simulink model "MOSSE_HDL_final"  (Simulink 8.3)
settings: Solver=FixedStepDiscrete  SolverMode=SingleTasking  StartTime=0.0  StopTime=30*640*360  RelTol=1e-3
InitFcn:
  | %% DSPBuilder Start
  | alt_dspbuilder_update_model(bdroot)
  | %% DSPBuilder End
  | param
StopFcn:
  | % r = rcount.Data(:,:);
  | % w = wcount.Data(:,:);
  | % d = dout.Data(:,:);
  | % ir = read.Data(:,:);
  | % iw = write.Data(:,:);
  | % z = double([ir iw d r w]');
  | %logic_analyzer
values from neighbouring files (symbols this model uses):
  Gau = [4035 -3983 3832 -3589 3269 -2890 2472 -2039 1612 -1211 854 -553 ... (4096 elements, 1x4096)]    [Gauss_coeff.mat]    (also in param.m = reshape(conj(Gau'), 1, 4096))
undefined symbols (not defined in the file or in its folder): gray, psr, source_1, source_2, State_Machine, State_Transition_Table1, window_hann
libraries: allblocks_alteradspbuilder2 x166, hdlsllib x24, hdldemolib x3, simulink x2, dspsigattribs x2, dspmtrx3 x2, visionsinks x1, visiontextngfix x1, dspvision x1
(part 3 of 4)

== system MOSSE_HDL_final/DSP_Builder_Compute_PSR/Std1 ==
  finish_flag : Inport
  demul_sel : Inport  Port=2
  Input_data : Inport  Port=3
  mean_ena : Inport  Port=4
  mean : Inport  Port=5
  std_count_ena : Inport  Port=6
  std_reset : Inport  Port=7
  Barrel Shifter : allblocks_alteradspbuilder2/Barrel Shifter  BusType=Signed Integer  bwl=44  bwr=8  pipeline=off  infer_distance=off  distance_length=4  ShiftDirection=Shift right  use_ena=off  use_aclr=off  UseDedicatedCircuitry=off  pipeline_display=0  allowFloatingPointOverride=on  logOutputs=off  logFile=d:\Project\AutoTracking\model\MOSSE_work\MOSSE_model\MOSSE_Final_models\tb_MOSSE_HDL_final\MOSSE%5FHDL%5Ffinal_DSP%5FBuilder%5FCompute%5FPSR_Std1_Barrel+Shifter.fixedpointlog
  Bitwise Logical Bus Operator : allblocks_alteradspbuilder2/Bitwise Logical Bus Operator  BusType=Unsigned Integer  bwl=1  bwr=0  LogicalOperator=AND  pipeline_display=0
  Constant1 : allblocks_alteradspbuilder2/Constant  mask_cst=0  BusType=Signed Integer  bwl=32  bwr=0  roundMode=Truncate  satMode=Wrap  SpecifyClock=off  allowFloatingPointOverride=on  logOutputs=off  logFile=d:\Project\AutoTracking\model\MOSSE_work\MOSSE_model\MOSSE_Final_models\tb_MOSSE_HDL_final\MOSSE%5FHDL%5Ffinal_DSP%5FBuilder%5FCompute%5FPSR_Std1_Constant1.fixedpointlog
  Constant2 : allblocks_alteradspbuilder2/Constant  mask_cst=12  BusType=Unsigned Integer  bwl=4  bwr=0  roundMode=Truncate  satMode=Wrap  SpecifyClock=off  allowFloatingPointOverride=on  logOutputs=off  logFile=d:\Project\AutoTracking\model\MOSSE_work\MOSSE_model\MOSSE_Final_models\tb_MOSSE_HDL_final\MOSSE%5FHDL%5Ffinal_DSP%5FBuilder%5FCompute%5FPSR_Std1_Constant2.fixedpointlog
  Delay1 : allblocks_alteradspbuilder2/Delay  pipeline=1  pipeline_display=1  ClockPhase=1  use_ena=off  use_sclr=off  allowFloatingPointOverride=on  logOutputs=off  logFile=d:\Project\AutoTracking\model\MOSSE_work\MOSSE_model\MOSSE_Final_models\tb_MOSSE_HDL_final\MOSSE%5FHDL%5Ffinal_DSP%5FBuilder%5FCompute%5FPSR_Std1_Delay1.fixedpointlog  use_init=off  reset_value=1
  Delay2 : allblocks_alteradspbuilder2/Delay  pipeline=1  pipeline_display=1  ClockPhase=1  use_ena=off  use_sclr=off  allowFloatingPointOverride=on  logOutputs=off  logFile=d:\Project\AutoTracking\model\MOSSE_work\MOSSE_model\MOSSE_Final_models\tb_MOSSE_HDL_final\MOSSE%5FHDL%5Ffinal_DSP%5FBuilder%5FCompute%5FPSR_Std1_Delay2.fixedpointlog  use_init=off  reset_value=1
  Multiplexer : allblocks_alteradspbuilder2/Multiplexer  numInputs=2  pipeline=0  oneHot=off  pipeline_display=0  use_ena=off  use_aclr=off  allowFloatingPointOverride=on  logOutputs=off  logFile=d:\Project\AutoTracking\model\MOSSE_work\MOSSE_model\MOSSE_Final_models\tb_MOSSE_HDL_final\MOSSE%5FHDL%5Ffinal_DSP%5FBuilder%5FCompute%5FPSR_Std1_Multiplexer.fixedpointlog
  Multiplexer2 : allblocks_alteradspbuilder2/Multiplexer  numInputs=2  pipeline=0  oneHot=off  pipeline_display=0  use_ena=off  use_aclr=off  allowFloatingPointOverride=on  logOutputs=off  logFile=d:\Project\AutoTracking\model\MOSSE_work\MOSSE_model\MOSSE_Final_models\tb_MOSSE_HDL_final\MOSSE%5FHDL%5Ffinal_DSP%5FBuilder%5FCompute%5FPSR_Std1_Multiplexer2.fixedpointlog
  Pipelined Adder : allblocks_alteradspbuilder2/Pipelined Adder  BusType=Signed Integer  bwl=32  bwr=0  pipeline=0  pipeline_display=0  AddSubDirection=SUB  use_cin=off  use_ovl=off  use_addsub=off  use_ena=off  use_aclr=off  or_aclr_inputs=on
  Pipelined Adder2 : allblocks_alteradspbuilder2/Pipelined Adder  BusType=Signed Integer  bwl=44  bwr=0  pipeline=1  pipeline_display=1  AddSubDirection=ADD  use_cin=off  use_ovl=off  use_addsub=off  use_ena=off  use_aclr=on  or_aclr_inputs=off
  Product : allblocks_alteradspbuilder2/Product  BusType=Signed Integer  bwl=32  bwr=0  pipeline=0  pipeline_display=0  phase_selection=1  use_ena=off  use_aclr=off  UseLPM=off  UseDedicatedCircuitry=on  allowFloatingPointOverride=on  logOutputs=off  logFile=d:\Project\AutoTracking\model\MOSSE_work\MOSSE_model\MOSSE_Final_models\tb_MOSSE_HDL_final\MOSSE%5FHDL%5Ffinal_DSP%5FBuilder%5FCompute%5FPSR_Std1_Product.fixedpointlog
  Square Root : allblocks_alteradspbuilder2/Square Root  BusType=Unsigned Integer  bwl=44  bwr=0  pipeline=0  pipeline_display=0  use_remain=off  use_ena=off  use_aclr=off
  Std_finish : Outport
  Std_val : Outport  Port=2
  wires:
  Pipelined Adder/1 -> Product/2, Product/1
  Product/1 -> Pipelined Adder2/1
  Constant2/1 -> Barrel Shifter/2
  Pipelined Adder2/1 -> Pipelined Adder2/2, Barrel Shifter/1
  Barrel Shifter/1 -> Square Root/1
  Square Root/1 -> Multiplexer2/3
  Input_data/1 -> Pipelined Adder/1
  demul_sel/1 -> Bitwise Logical Bus Operator/2
  finish_flag/1 -> Bitwise Logical Bus Operator/1
  Delay1/1 -> Std_finish/1
  Constant1/1 -> Multiplexer/2
  mean_ena/1 -> Multiplexer/1
  mean/1 -> Multiplexer/3
  Multiplexer/1 -> Pipelined Adder/2
  std_count_ena/1 -> Multiplexer2/1
  Multiplexer2/1 -> Delay2/1
  Delay2/1 -> Std_val/1, Multiplexer2/2
  Bitwise Logical Bus Operator/1 -> Delay1/1
  std_reset/1 -> Pipelined Adder2/3

== system MOSSE_HDL_final/DSP_Builder_Compute_PSR/Vals_gen ==
  count_ena : Inport
  counter : Inport  Port=2
  demul_sel : Inport  Port=3
  Constant2 : allblocks_alteradspbuilder2/Constant  mask_cst=0  BusType=Single Bit  bwl=16  bwr=0  roundMode=Truncate  satMode=Wrap  SpecifyClock=off  allowFloatingPointOverride=on  logOutputs=off  logFile=d:\Project\AutoTracking\model\MOSSE_work\MOSSE_model\MOSSE_Final_models\tb_MOSSE_HDL_final\MOSSE%5FHDL%5Ffinal_DSP%5FBuilder%5FCompute%5FPSR_Vals%5Fgen_Constant2.fixedpointlog
  Demultiplexer : allblocks_alteradspbuilder2/Demultiplexer  numOutputs=2  pipeline_display=1  use_ena=off  use_sclr=off  allowFloatingPointOverride=on  logOutputs=off  logFile=d:\Project\AutoTracking\model\MOSSE_work\MOSSE_model\MOSSE_Final_models\tb_MOSSE_HDL_final\MOSSE%5FHDL%5Ffinal_DSP%5FBuilder%5FCompute%5FPSR_Vals%5Fgen_Demultiplexer%3A%3Aq.fixedpointlog,d:\Project\AutoTracking\model\MOSSE_work\MOSSE_model\MOSSE_Final_models\tb_MOSSE_HDL_final\MOSSE%5FHDL%5Ffinal_DSP%5FBuilder%5FCompute%5FPSR_Vals%5Fgen_Demultiplexer%3A%3Aq.fixedpointlog,
  Multiplexer : allblocks_alteradspbuilder2/Multiplexer  numInputs=2  pipeline=0  oneHot=off  pipeline_display=0  use_ena=off  use_aclr=off  allowFloatingPointOverride=on  logOutputs=off  logFile=d:\Project\AutoTracking\model\MOSSE_work\MOSSE_model\MOSSE_Final_models\tb_MOSSE_HDL_final\MOSSE%5FHDL%5Ffinal_DSP%5FBuilder%5FCompute%5FPSR_Vals%5Fgen_Multiplexer.fixedpointlog
  1_channel : Outport
  2_channel : Outport  Port=2
  wires:
  Multiplexer/1 -> Demultiplexer/1
  Demultiplexer/1 -> 1_channel/1
  Demultiplexer/2 -> 2_channel/1
  demul_sel/1 -> Demultiplexer/2
  Constant2/1 -> Multiplexer/2
  counter/1 -> Multiplexer/3
  count_ena/1 -> Multiplexer/1

== system MOSSE_HDL_final/DSP_Builder_Mult_complex/Gauss_table ==
  rst : Inport
  enb : Inport  Port=2
  Counter : allblocks_alteradspbuilder2/Counter  BusType=Unsigned Integer  bwl=12  bwr=0  use_modulo=off  modulo=255  SpecifyClock=off  direction=Increment  use_sload=off  use_sset=off  svalue=1  use_clk_ena=off  use_ena=on  use_sclr=on  pipeline_display=1
  ROM : allblocks_alteradspbuilder2/ROM  numwords=4096  BusType=Signed Integer  bwl=16  bwr=0  memory_type=AUTO  ram_type=ROM  initialization=From MATLAB array  init_file=input.hex  init_array=imag(Gau)  register_outputs=off  use_ena=off  ClockPhase=1  pipeline_display=1  allowFloatingPointOverride=on  logOutputs=off  logFile=E:\Work\ComputerVision\ObjectTrack\MOSSE\autotrackigproject\Model\MOSSE_algorithm\MOSSE_simulink\tb_MOSSE_HDL_final\MOSSE%5FHDL%5Ffinal_DSP%5FBuilder%5FMult%5Fcomplex_Gauss%5Ftable_ROM.fixedpointlog  enable_runtime_mod=off  instance_name=AAAA
  ROM1 : allblocks_alteradspbuilder2/ROM  numwords=4096  BusType=Signed Integer  bwl=16  bwr=0  memory_type=AUTO  ram_type=ROM  initialization=From MATLAB array  init_file=input.hex  init_array=real(Gau)  register_outputs=off  use_ena=off  ClockPhase=1  pipeline_display=1  allowFloatingPointOverride=on  logOutputs=off  logFile=E:\Work\ComputerVision\ObjectTrack\MOSSE\autotrackigproject\Model\MOSSE_algorithm\MOSSE_simulink\tb_MOSSE_HDL_final\MOSSE%5FHDL%5Ffinal_DSP%5FBuilder%5FMult%5Fcomplex_Gauss%5Ftable_ROM1.fixedpointlog  enable_runtime_mod=off  instance_name=AAAA
  Coeff_real : Outport
  Coeff_imag : Outport  Port=2
  wires:
  Counter/1 -> ROM/1, ROM1/1
  ROM1/1 -> Coeff_real/1
  ROM/1 -> Coeff_imag/1
  rst/1 -> Counter/2
  enb/1 -> Counter/1

== system MOSSE_HDL_final/HDL_CODER_Subsystem/Comp_Shift_code_Subsys ==
  Max_num : Inport
  iaclr : Inport  Port=2
  Comp_Shift_code : MATLAB Function
  dx : Outport
  dy : Outport  Port=2
  wires:
  Comp_Shift_code/2(dy) -> dy/1
  Comp_Shift_code/1(dx) -> dx/1
  Max_num/1 -> Comp_Shift_code/2(max_num)
  iaclr/1 -> Comp_Shift_code/1(iaclr)

== system MOSSE_HDL_final/HDL_CODER_Subsystem/Complex_2_real_imag ==
  H1 : Inport
  H2 : Inport  Port=2
  Complex to Real-Imag_H1 : ComplexToRealImag
  Complex to Real-Imag_H2 : ComplexToRealImag
  Terminator : Terminator
  Real_H1 : Outport
  Real_H2 : Outport  Port=2
  Imag_H1 : Outport  Port=3
  wires:
  Complex to Real-Imag_H2/2 -> Terminator/1
  Complex to Real-Imag_H1/1 -> Real_H1/1
  Complex to Real-Imag_H2/1 -> Real_H2/1
  Complex to Real-Imag_H1/2 -> Imag_H1/1
  H2/1 -> Complex to Real-Imag_H2/1
  H1/1 -> Complex to Real-Imag_H1/1

== system MOSSE_HDL_final/HDL_CODER_Subsystem/FFT2D_System ==
  en_R : Inport
  read_R : Inport  Port=2
  write_R : Inport  Port=3
  iData : Inport  Port=4
  iMux_mult : Inport  Port=5
  Corr_Data : Inport  Port=6
  Mux : Inport  Port=7
  image : Inport  Port=8
  Start : Inport  Port=9
  Enb : Inport  Port=10
  FFT2D_System : Subsystem
  Mux_Mult : Subsystem
  R_RAM : Subsystem
  F* : Outport
  F : Outport  Port=2
  IFFT_res : Outport  Port=3
  data_ready : Outport  Port=4
  end : Outport  Port=5
  wires:
  en_R/1 -> R_RAM/1(en_m)
  read_R/1 -> R_RAM/2(read_m)
  write_R/1 -> R_RAM/3(write_m)
  R_RAM/1(oData) -> FFT2D_System/1(Input1)
  image/1 -> FFT2D_System/3(Input2)
  Mux/1 -> FFT2D_System/2(Mux)
  Start/1 -> FFT2D_System/4(Start)
  Enb/1 -> FFT2D_System/5(Enb)
  FFT2D_System/2(data_ready) -> data_ready/1
  FFT2D_System/3(end) -> end/1
  iMux_mult/1 -> Mux_Mult/1(iMux_muLt)
  Corr_Data/1 -> Mux_Mult/2(Corr)
  FFT2D_System/1(oFFT2) -> Mux_Mult/3(iData)
  Mux_Mult/1(F*) -> F*/1
  Mux_Mult/2(F) -> F/1
  Mux_Mult/3(IFFT_res) -> IFFT_res/1
  iData/1 -> R_RAM/4(iData)

== system MOSSE_HDL_final/HDL_CODER_Subsystem/IFFT_MUX ==
  IFFT_res : Inport
  Mux : Inport  Port=2
  IFFT_res1 : Inport  Port=3
  Complex to Real-Imag2 : ComplexToRealImag  Output=Real  SampleTime=1
  Data Type Conversion2 : DataTypeConversion  OutDataTypeStr=int16
  IFFT_div : hdlsllib/HDL Operations/Bit Shift  mode=Shift Right Arithmetic  N=12
  IFFT_ress_mult : MultiPortSwitch  DataPortOrder=Zero-based contiguous  Inputs=2  zeroidx=on  SampleTime=1
  RAM_data : Outport
  oData : Outport  Port=2
  wires:
  Complex to Real-Imag2/1 -> IFFT_div/1
  IFFT_res1/1 -> IFFT_ress_mult/3
  Data Type Conversion2/1 -> RAM_data/1, IFFT_ress_mult/2
  IFFT_ress_mult/1 -> oData/1
  Mux/1 -> IFFT_ress_mult/1
  IFFT_div/1 -> Data Type Conversion2/1
  IFFT_res/1 -> Complex to Real-Imag2/1

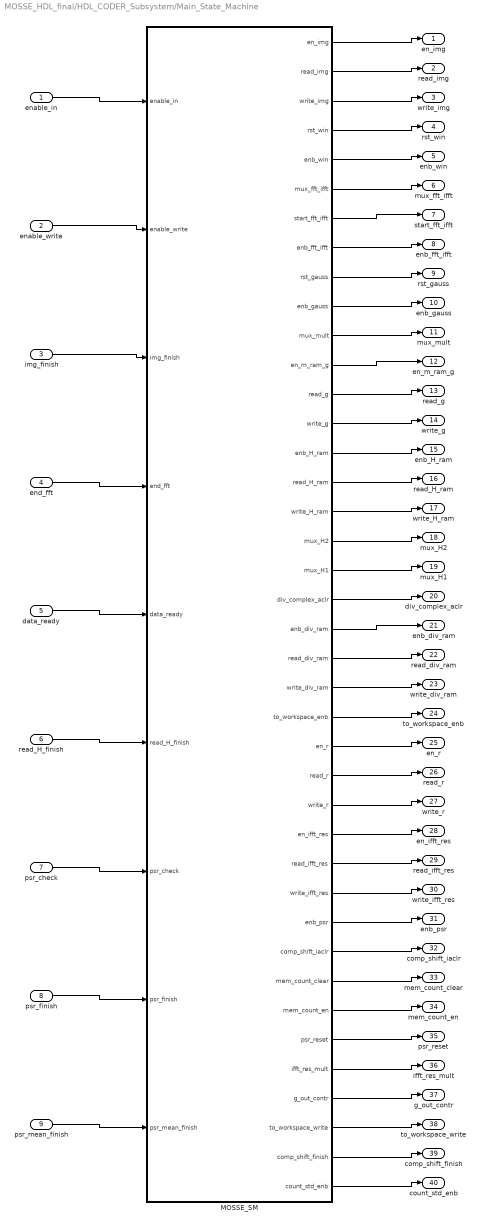
== system MOSSE_HDL_final/HDL_CODER_Subsystem/Main_State_Machine ==
  enable_in : Inport
  enable_write : Inport  Port=2
  img_finish : Inport  Port=3
  end_fft : Inport  Port=4
  data_ready : Inport  Port=5
  read_H_finish : Inport  Port=6
  psr_check : Inport  Port=7
  psr_finish : Inport  Port=8
  psr_mean_finish : Inport  Port=9
  MOSSE_SM : State Transition Table  TreatAsAtomicUnit=on
  en_img : Outport
  read_img : Outport  Port=2
  write_img : Outport  Port=3
  rst_win : Outport  Port=4
  enb_win : Outport  Port=5
  mux_fft_ifft : Outport  Port=6
  start_fft_ifft : Outport  Port=7
  enb_fft_ifft : Outport  Port=8
  rst_gauss : Outport  Port=9
  enb_gauss : Outport  Port=10
  mux_mult : Outport  Port=11
  en_m_ram_g : Outport  Port=12
  read_g : Outport  Port=13
  write_g : Outport  Port=14
  enb_H_ram : Outport  Port=15
  read_H_ram : Outport  Port=16
  write_H_ram : Outport  Port=17
  mux_H2 : Outport  Port=18
  mux_H1 : Outport  Port=19
  div_complex_aclr : Outport  Port=20
  enb_div_ram : Outport  Port=21
  read_div_ram : Outport  Port=22
  write_div_ram : Outport  Port=23
  to_workspace_enb : Outport  Port=24
  en_r : Outport  Port=25
  read_r : Outport  Port=26
  write_r : Outport  Port=27
  en_ifft_res : Outport  Port=28
  read_ifft_res : Outport  Port=29
  write_ifft_res : Outport  Port=30
  enb_psr : Outport  Port=31
  comp_shift_iaclr : Outport  Port=32
  mem_count_clear : Outport  Port=33
  mem_count_en : Outport  Port=34
  psr_reset : Outport  Port=35
  ifft_res_mult : Outport  Port=36
  g_out_contr : Outport  Port=37
  to_workspace_write : Outport  Port=38
  comp_shift_finish : Outport  Port=39
  count_std_enb : Outport  Port=40
  wires:
  MOSSE_SM/24(to_workspace_enb) -> to_workspace_enb/1
  MOSSE_SM/10(enb_gauss) -> enb_gauss/1
  MOSSE_SM/7(start_fft_ifft) -> start_fft_ifft/1
  MOSSE_SM/2(read_img) -> read_img/1
  MOSSE_SM/11(mux_mult) -> mux_mult/1
  MOSSE_SM/15(enb_H_ram) -> enb_H_ram/1
  img_finish/1 -> MOSSE_SM/3(img_finish)
  MOSSE_SM/6(mux_fft_ifft) -> mux_fft_ifft/1
  data_ready/1 -> MOSSE_SM/5(data_ready)
  MOSSE_SM/8(enb_fft_ifft) -> enb_fft_ifft/1
  MOSSE_SM/12(en_m_ram_g) -> en_m_ram_g/1
  MOSSE_SM/17(write_H_ram) -> write_H_ram/1
  MOSSE_SM/18(mux_H2) -> mux_H2/1
  MOSSE_SM/14(write_g) -> write_g/1
  MOSSE_SM/16(read_H_ram) -> read_H_ram/1
  enable_in/1 -> MOSSE_SM/1(enable_in)
  MOSSE_SM/13(read_g) -> read_g/1
  MOSSE_SM/4(rst_win) -> rst_win/1
  MOSSE_SM/5(enb_win) -> enb_win/1
  end_fft/1 -> MOSSE_SM/4(end_fft)
  MOSSE_SM/3(write_img) -> write_img/1
  MOSSE_SM/9(rst_gauss) -> rst_gauss/1
  MOSSE_SM/22(read_div_ram) -> read_div_ram/1
  MOSSE_SM/19(mux_H1) -> mux_H1/1
  MOSSE_SM/23(write_div_ram) -> write_div_ram/1
  MOSSE_SM/21(enb_div_ram) -> enb_div_ram/1
  MOSSE_SM/20(div_complex_aclr) -> div_complex_aclr/1
  read_H_finish/1 -> MOSSE_SM/6(read_H_finish)
  MOSSE_SM/25(en_r) -> en_r/1
  MOSSE_SM/1(en_img) -> en_img/1
  MOSSE_SM/26(read_r) -> read_r/1
  MOSSE_SM/27(write_r) -> write_r/1
  MOSSE_SM/28(en_ifft_res) -> en_ifft_res/1
  MOSSE_SM/29(read_ifft_res) -> read_ifft_res/1
  MOSSE_SM/34(mem_count_en) -> mem_count_en/1
  MOSSE_SM/31(enb_psr) -> enb_psr/1
  MOSSE_SM/30(write_ifft_res) -> write_ifft_res/1
  MOSSE_SM/32(comp_shift_iaclr) -> comp_shift_iaclr/1
  MOSSE_SM/33(mem_count_clear) -> mem_count_clear/1
  MOSSE_SM/36(ifft_res_mult) -> ifft_res_mult/1
  psr_check/1 -> MOSSE_SM/7(psr_check)
  psr_finish/1 -> MOSSE_SM/8(psr_finish)
  psr_mean_finish/1 -> MOSSE_SM/9(psr_mean_finish)
  MOSSE_SM/35(psr_reset) -> psr_reset/1
  MOSSE_SM/37(g_out_contr) -> g_out_contr/1
  enable_write/1 -> MOSSE_SM/2(enable_write)
  MOSSE_SM/38(to_workspace_write) -> to_workspace_write/1
  MOSSE_SM/39(comp_shift_finish) -> comp_shift_finish/1
  MOSSE_SM/40(count_std_enb) -> count_std_enb/1

== system MOSSE_HDL_final/HDL_CODER_Subsystem/Memory_Counter_Subsys ==
  dx : Inport
  dy : Inport  Port=2
  clear : Inport  Port=3
  en : Inport  Port=4
  Memory Counter : MATLAB Function
  addr : Outport
  wires:
  dy/1 -> Memory Counter/4(dy)
  en/1 -> Memory Counter/2(en)
  dx/1 -> Memory Counter/3(dx)
  clear/1 -> Memory Counter/1(clear)
  Memory Counter/1(count) -> addr/1

== system MOSSE_HDL_final/HDL_CODER_Subsystem/Mux_system ==
  iMux_Mult : Inport
  iData1 : Inport  Port=2
  iData2 : Inport  Port=3
  iH1_1 : Inport  Port=4
  iMux_H1 : Inport  Port=5
  iH1_2 : Inport  Port=6
  iMux_H2 : Inport  Port=7
  iH2_2 : Inport  Port=8
  iH2_1 : Inport  Port=9
  Delay2 : Delay  DelayLength=1  InitialCondition=0
  Delay3 : Delay  DelayLength=1  InitialCondition=0
  Mux_H1 : MultiPortSwitch  DataPortOrder=Zero-based contiguous  Inputs=2  zeroidx=on  SampleTime=1
  Mux_H2 : MultiPortSwitch  DataPortOrder=Zero-based contiguous  Inputs=2  zeroidx=on  SampleTime=1
  Mux_Mult1 : MultiPortSwitch  DataPortOrder=Zero-based contiguous  Inputs=2  zeroidx=on  SampleTime=1
  Mux_Mult2 : MultiPortSwitch  DataPortOrder=Zero-based contiguous  Inputs=2  zeroidx=on  SampleTime=1
  H2 : Outport
  H1 : Outport  Port=2
  oData1 : Outport  Port=3
  oData2 : Outport  Port=4
  wires:
  iH2_2/1 -> Mux_H2/3
  iH1_2/1 -> Mux_H1/3
  iMux_H2/1 -> Mux_H2/1
  iMux_H1/1 -> Mux_H1/1
  Mux_Mult1/1 -> oData1/1
  Mux_Mult2/1 -> oData2/1
  iData1/1 -> Delay3/1, Mux_Mult1/2
  Delay3/1 -> Mux_Mult1/3
  iData2/1 -> Mux_Mult2/2, Delay2/1
  Delay2/1 -> Mux_Mult2/3
  iMux_Mult/1 -> Mux_Mult1/1, Mux_Mult2/1
  Mux_H1/1 -> H1/1
  Mux_H2/1 -> H2/1
  iH1_1/1 -> Mux_H1/2
  iH2_1/1 -> Mux_H2/2

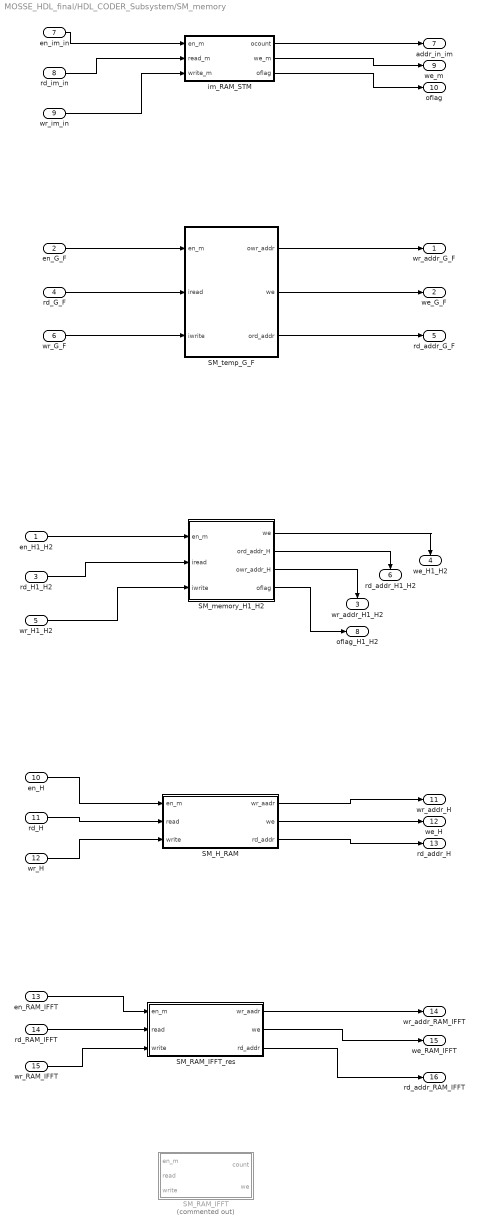
== system MOSSE_HDL_final/HDL_CODER_Subsystem/SM_memory ==
  en_H1_H2 : Inport
  en_G_F : Inport  Port=2
  rd_H1_H2 : Inport  Port=3
  rd_G_F : Inport  Port=4
  wr_H1_H2 : Inport  Port=5
  wr_G_F : Inport  Port=6
  en_im_in : Inport  Port=7
  rd_im_in : Inport  Port=8
  wr_im_in : Inport  Port=9
  en_H : Inport  Port=10
  rd_H : Inport  Port=11
  wr_H : Inport  Port=12
  en_RAM_IFFT : Inport  Port=13
  rd_RAM_IFFT : Inport  Port=14
  wr_RAM_IFFT : Inport  Port=15
  SM_H_RAM : Subsystem
  SM_RAM_IFFT : Subsystem  Commented=on
  SM_RAM_IFFT_res : Subsystem
  SM_memory_H1_H2 : Subsystem
  SM_temp_G_F : Subsystem
  im_RAM_STM : Subsystem
  wr_addr_G_F : Outport
  we_G_F : Outport  Port=2
  wr_addr_H1_H2 : Outport  Port=3
  we_H1_H2 : Outport  Port=4
  rd_addr_G_F : Outport  Port=5
  rd_addr_H1_H2 : Outport  Port=6
  addr_in_im : Outport  Port=7
  oflag_H1_H2 : Outport  Port=8
  we_m : Outport  Port=9
  oflag : Outport  Port=10
  wr_addr_H : Outport  Port=11
  we_H : Outport  Port=12
  rd_addr_H : Outport  Port=13
  wr_addr_RAM_IFFT : Outport  Port=14
  we_RAM_IFFT : Outport  Port=15
  rd_addr_RAM_IFFT : Outport  Port=16
  wires:
  en_im_in/1 -> im_RAM_STM/1(en_m)
  rd_im_in/1 -> im_RAM_STM/2(read_m)
  wr_im_in/1 -> im_RAM_STM/3(write_m)
  im_RAM_STM/1(ocount) -> addr_in_im/1
  im_RAM_STM/2(we_m) -> we_m/1
  im_RAM_STM/3(oflag) -> oflag/1
  en_RAM_IFFT/1 -> SM_RAM_IFFT_res/1(en_m)
  rd_RAM_IFFT/1 -> SM_RAM_IFFT_res/2(read)
  wr_RAM_IFFT/1 -> SM_RAM_IFFT_res/3(write)
  SM_RAM_IFFT_res/1(wr_aadr) -> wr_addr_RAM_IFFT/1
  SM_RAM_IFFT_res/2(we) -> we_RAM_IFFT/1
  en_H/1 -> SM_H_RAM/1(en_m)
  rd_H/1 -> SM_H_RAM/2(read)
  wr_H/1 -> SM_H_RAM/3(write)
  SM_H_RAM/1(wr_aadr) -> wr_addr_H/1
  SM_H_RAM/2(we) -> we_H/1
  SM_H_RAM/3(rd_addr) -> rd_addr_H/1
  SM_memory_H1_H2/1(we) -> we_H1_H2/1
  SM_memory_H1_H2/3(owr_addr_H) -> wr_addr_H1_H2/1
  SM_memory_H1_H2/2(ord_addr_H) -> rd_addr_H1_H2/1
  en_H1_H2/1 -> SM_memory_H1_H2/1(en_m)
  rd_H1_H2/1 -> SM_memory_H1_H2/2(iread)
  wr_H1_H2/1 -> SM_memory_H1_H2/3(iwrite)
  SM_memory_H1_H2/4(oflag) -> oflag_H1_H2/1
  SM_temp_G_F/3(ord_addr) -> rd_addr_G_F/1
  SM_temp_G_F/2(we) -> we_G_F/1
  SM_temp_G_F/1(owr_addr) -> wr_addr_G_F/1
  en_G_F/1 -> SM_temp_G_F/1(en_m)
  rd_G_F/1 -> SM_temp_G_F/2(iread)
  wr_G_F/1 -> SM_temp_G_F/3(iwrite)
  SM_RAM_IFFT_res/3(rd_addr) -> rd_addr_RAM_IFFT/1

== system MOSSE_HDL_final/HDL_CODER_Subsystem/psr_code_subsys ==
  enb : Inport
  rst : Inport  Port=2
  idata : Inport  Port=3
  count_std_enb : Inport  Port=4
  Compute_PSR_code : MATLAB Function
  counter : Outport
  max_index : Outport  Port=2
  max_value : Outport  Port=3
  mean_value : Outport  Port=4
  mean_finish : Outport  Port=5
  psr_finish : Outport  Port=6
  std_value : Outport  Port=7
  wires:
  Compute_PSR_code/6(mean_finish) -> mean_finish/1
  Compute_PSR_code/1(counter) -> counter/1
  Compute_PSR_code/4(mean_value) -> mean_value/1
  Compute_PSR_code/5(std_value) -> std_value/1
  Compute_PSR_code/2(max_index) -> max_index/1
  Compute_PSR_code/3(max_value) -> max_value/1
  Compute_PSR_code/7(psr_finish) -> psr_finish/1
  enb/1 -> Compute_PSR_code/1(enb)
  rst/1 -> Compute_PSR_code/2(rst)
  idata/1 -> Compute_PSR_code/3(idata)
  count_std_enb/1 -> Compute_PSR_code/4(count_std_enb)

== system MOSSE_HDL_final/Source/source_1 ==
  In1 : Inport
  Enable : EnablePort
  source_1 : LookupNDDirect  NumberOfTableDimensions=1  Table=source_1  TableDataTypeStr=int16
  Out1 : Outport
  wires:
  source_1/1 -> Out1/1
  In1/1 -> source_1/1

== system MOSSE_HDL_final/Source/source_2 ==
  In1 : Inport
  Enable : EnablePort
  source_2 : LookupNDDirect  NumberOfTableDimensions=1  Table=source_2  TableDataTypeStr=int16
  Out1 : Outport
  wires:
  source_2/1 -> Out1/1
  In1/1 -> source_2/1

== system MOSSE_HDL_final/Video_TestBench/Write_control_subsys ==
  addr_x : Inport
  addr_y : Inport  Port=2
  dx : Inport  Port=3
  dy : Inport  Port=4
  x_init : Inport  Port=5
  y_init : Inport  Port=6
  comp_shift_finish : Inport  Port=7
  Write_control_STM : State Transition Table  TreatAsAtomicUnit=on
  x_coord : Outport
  y_coord : Outport  Port=2
  enable_write : Outport  Port=3
  to_workspace_enb : Outport  Port=4
  frame_num : Outport  Port=5
  wires:
  x_init/1 -> Write_control_STM/6(x_init)
  y_init/1 -> Write_control_STM/7(y_init)
  dx/1 -> Write_control_STM/3(dx)
  dy/1 -> Write_control_STM/4(dy)
  Write_control_STM/1(x_coord) -> x_coord/1
  Write_control_STM/3(enable_write) -> enable_write/1
  Write_control_STM/2(y_coord) -> y_coord/1
  comp_shift_finish/1 -> Write_control_STM/5(comp_shift_finish)
  Write_control_STM/4(to_workspace_enable) -> to_workspace_enb/1
  addr_x/1 -> Write_control_STM/1(addr_x)
  addr_y/1 -> Write_control_STM/2(addr_y)
  Write_control_STM/5(frame_num) -> frame_num/1

== system MOSSE_HDL_final/Video_TestBench/deserialize1 ==
  serialin : Inport
  Buffer : Buffer  N=640*360  TreatMby1Signals=One channel
  Convert 1-D to 2-D : dspsigattribs/Convert 1-D to 2-D  M=640  N=360  frameBasedOut=off
  Frame Conversion : FrameConversion  OutFrame=Sample-based
  Transpose : dspmtrx3/Transpose  Hermitian=off  overflowFlag=on
  imgout : Outport
  wires:
  Buffer/1 -> Frame Conversion/1
  serialin/1 -> Buffer/1
  Convert 1-D to 2-D/1 -> Transpose/1
  Frame Conversion/1 -> Convert 1-D to 2-D/1
  Transpose/1 -> imgout/1

== system MOSSE_HDL_final/Video_TestBench/serialize ==
  img : Inport
  Convert 2-D to 1-D : dspsigattribs/Convert 2-D to 1-D
  Frame Conversion : FrameConversion
  Transpose : dspmtrx3/Transpose  Hermitian=off  overflowFlag=on
  Unbuffer : Unbuffer  SampleBasedProcessing=Same as frame based
  serial : Outport  SampleTime=1
  wires:
  Convert 2-D to 1-D/1 -> Frame Conversion/1
  img/1 -> Transpose/1
  Transpose/1 -> Convert 2-D to 1-D/1
  Frame Conversion/1 -> Unbuffer/1
  Unbuffer/1 -> serial/1

== system MOSSE_HDL_final/HDL_CODER_Subsystem/FFT2D_System/FFT2D_System ==
  Input1 : Inport
  Mux : Inport  Port=2
  Input2 : Inport  Port=3
  Start : Inport  Port=4
  Enb : Inport  Port=5
  Data Type Conversion1 : DataTypeConversion  OutDataTypeStr=fixdt(1,24,0)
  FFT/IFTT Mux : MultiPortSwitch  DataPortOrder=Zero-based contiguous  Inputs=2  zeroidx=on  OutDataTypeStr=fixdt(1,24,0)  SampleTime=1
  FFT2D/IFFT2D : Subsystem
  Real-Imag to Complex1 : RealImagToComplex  Input=Real  SampleTime=1
  oFFT2 : Outport
  data_ready : Outport  Port=2
  end : Outport  Port=3
  wires:
  FFT/IFTT Mux/1 -> FFT2D/IFFT2D/1(input)
  FFT2D/IFFT2D/3(end) -> end/1
  FFT2D/IFFT2D/1(oFFT2) -> oFFT2/1
  Input2/1 -> Data Type Conversion1/1
  Mux/1 -> FFT/IFTT Mux/1
  Enb/1 -> FFT2D/IFFT2D/3(Enb)
  Input1/1 -> FFT/IFTT Mux/2
  Data Type Conversion1/1 -> Real-Imag to Complex1/1
  Start/1 -> FFT2D/IFFT2D/2(Start)
  FFT2D/IFFT2D/2(data_ready) -> data_ready/1
  Real-Imag to Complex1/1 -> FFT/IFTT Mux/3

== system MOSSE_HDL_final/HDL_CODER_Subsystem/FFT2D_System/Mux_Mult ==
  iMux_muLt : Inport
  Corr : Inport  Port=2
  iData : Inport  Port=3
  Complex to Real-Imag : ComplexToRealImag
  Data Type Conversion3 : DataTypeConversion  OutDataTypeStr=int32
  Math Function1 : Math  Operator=conj  SaturateOnIntegerOverflow=on
  Mux_Mult : MultiPortSwitch  DataPortOrder=Zero-based contiguous  Inputs=2  zeroidx=on  SampleTime=1
  Real-Imag to Complex : RealImagToComplex
  Window_div1 : hdlsllib/HDL Operations/Bit Shift  mode=Shift Right Arithmetic  N=3
  Window_div2 : hdlsllib/HDL Operations/Bit Shift  mode=Shift Right Arithmetic  N=3
  F* : Outport
  F : Outport  Port=2
  IFFT_res : Outport  Port=3
  wires:
  Corr/1 -> Mux_Mult/3
  Math Function1/1 -> Mux_Mult/2
  iMux_muLt/1 -> Mux_Mult/1
  Data Type Conversion3/1 -> Complex to Real-Imag/1, IFFT_res/1
  Mux_Mult/1 -> F*/1
  iData/1 -> Data Type Conversion3/1
  Complex to Real-Imag/2 -> Window_div2/1
  Complex to Real-Imag/1 -> Window_div1/1
  Real-Imag to Complex/1 -> F/1, Math Function1/1
  Window_div1/1 -> Real-Imag to Complex/1
  Window_div2/1 -> Real-Imag to Complex/2

== system MOSSE_HDL_final/HDL_CODER_Subsystem/FFT2D_System/R_RAM ==
  en_m : Inport
  read_m : Inport  Port=2
  write_m : Inport  Port=3
  iData : Inport  Port=4
  Data Type Conversion : DataTypeConversion  OutDataTypeStr=fixdt(1,24,0)
  Math Function : Math  Operator=conj  SaturateOnIntegerOverflow=on
  Read_Write_SM6 : State Transition Table  TreatAsAtomicUnit=on
  Simple Dual Port RAM : hdlsllib/HDL Operations/Simple Dual Port RAM  ram_size=12
  WRADDR_R : hdlsllib/HDL Operations/HDL Counter  CountType=Free running  CountInit=0  CountStep=1  CountMax=100  CountFromType=Initial value  CountFrom=0  CountResetPort=on  CountLoadPort=off  CountEnbPort=on  CountDirPort=off  CountDataType=Unsigned  CountWordLen=12  CountFracLen=0  CountSampTime=1
  oData : Outport
  wires:
  Read_Write_SM6/3(enb_img) -> WRADDR_R/2
  write_m/1 -> Read_Write_SM6/3(write)
  en_m/1 -> Read_Write_SM6/1(en_m)
  read_m/1 -> Read_Write_SM6/2(read)
  Simple Dual Port RAM/1 -> oData/1
  Read_Write_SM6/2(rst_img) -> WRADDR_R/1
  Math Function/1 -> Data Type Conversion/1
  iData/1 -> Math Function/1
  Data Type Conversion/1 -> Simple Dual Port RAM/1
  WRADDR_R/1 -> Simple Dual Port RAM/4, Simple Dual Port RAM/2
  Read_Write_SM6/1(we) -> Simple Dual Port RAM/3

== system MOSSE_HDL_final/HDL_CODER_Subsystem/SM_memory/SM_H_RAM ==
  en_m : Inport
  read : Inport  Port=2
  write : Inport  Port=3
  RADDR_H2 : hdlsllib/HDL Operations/HDL Counter  CountType=Free running  CountInit=0  CountStep=1  CountMax=100  CountFromType=Initial value  CountFrom=0  CountResetPort=on  CountLoadPort=off  CountEnbPort=on  CountDirPort=off  CountDataType=Unsigned  CountWordLen=12  CountFracLen=0  CountSampTime=1
  Read_Write_SM1_patched_2 : State Transition Table  TreatAsAtomicUnit=on
  WADDR_H2 : hdlsllib/HDL Operations/HDL Counter  CountType=Free running  CountInit=0  CountStep=1  CountMax=100  CountFromType=Initial value  CountFrom=0  CountResetPort=on  CountLoadPort=off  CountEnbPort=on  CountDirPort=off  CountDataType=Unsigned  CountWordLen=12  CountFracLen=0  CountSampTime=1
  wr_aadr : Outport
  we : Outport  Port=2
  rd_addr : Outport  Port=3
  wires:
  RADDR_H2/1 -> rd_addr/1
  Read_Write_SM1_patched_2/2(rst_r) -> RADDR_H2/1
  Read_Write_SM1_patched_2/3(enb_r) -> RADDR_H2/2
  Read_Write_SM1_patched_2/5(enb_w) -> WADDR_H2/2
  Read_Write_SM1_patched_2/4(rst_w) -> WADDR_H2/1
  read/1 -> Read_Write_SM1_patched_2/2(read)
  Read_Write_SM1_patched_2/1(we) -> we/1
  en_m/1 -> Read_Write_SM1_patched_2/1(en_m)
  write/1 -> Read_Write_SM1_patched_2/3(write)
  WADDR_H2/1 -> wr_aadr/1

== system MOSSE_HDL_final/HDL_CODER_Subsystem/SM_memory/SM_RAM_IFFT ==
  en_m : Inport
  read : Inport  Port=2
  write : Inport  Port=3
  IFFT_counter : hdldemolib/HDL Counter  CountType=Free running  CountInit=0  CountStep=1  CountMax=100  CountFromType=Initial value  CountFrom=0  CountResetPort=on  CountLoadPort=off  CountEnbPort=on  CountDirPort=off  CountDataType=Unsigned  CountWordLen=12  CountFracLen=0  CountSampTime=1
  Read_Write_SM7 : State Transition Table  TreatAsAtomicUnit=on
  count : Outport
  we : Outport  Port=2
  wires:
  IFFT_counter/1 -> count/1
  Read_Write_SM7/2(rst_img) -> IFFT_counter/1
  Read_Write_SM7/3(enb_img) -> IFFT_counter/2
  Read_Write_SM7/1(we) -> we/1
  read/1 -> Read_Write_SM7/2(read)
  write/1 -> Read_Write_SM7/3(write)
  en_m/1 -> Read_Write_SM7/1(en_m)

== system MOSSE_HDL_final/HDL_CODER_Subsystem/SM_memory/SM_RAM_IFFT_res ==
  en_m : Inport
  read : Inport  Port=2
  write : Inport  Port=3
  RADDR_H2 : hdlsllib/HDL Operations/HDL Counter  CountType=Free running  CountInit=0  CountStep=1  CountMax=100  CountFromType=Initial value  CountFrom=0  CountResetPort=on  CountLoadPort=off  CountEnbPort=on  CountDirPort=off  CountDataType=Unsigned  CountWordLen=12  CountFracLen=0  CountSampTime=1
  Read_Write_SM1_patched_2 : State Transition Table  TreatAsAtomicUnit=on
  WADDR_H2 : hdlsllib/HDL Operations/HDL Counter  CountType=Free running  CountInit=0  CountStep=1  CountMax=100  CountFromType=Initial value  CountFrom=0  CountResetPort=on  CountLoadPort=off  CountEnbPort=on  CountDirPort=off  CountDataType=Unsigned  CountWordLen=12  CountFracLen=0  CountSampTime=1
  wr_aadr : Outport
  we : Outport  Port=2
  rd_addr : Outport  Port=3
  wires:
  RADDR_H2/1 -> rd_addr/1
  Read_Write_SM1_patched_2/2(rst_r) -> RADDR_H2/1
  Read_Write_SM1_patched_2/3(enb_r) -> RADDR_H2/2
  Read_Write_SM1_patched_2/5(enb_w) -> WADDR_H2/2
  Read_Write_SM1_patched_2/4(rst_w) -> WADDR_H2/1
  read/1 -> Read_Write_SM1_patched_2/2(read)
  Read_Write_SM1_patched_2/1(we) -> we/1
  en_m/1 -> Read_Write_SM1_patched_2/1(en_m)
  write/1 -> Read_Write_SM1_patched_2/3(write)
  WADDR_H2/1 -> wr_aadr/1

== system MOSSE_HDL_final/HDL_CODER_Subsystem/SM_memory/SM_memory_H1_H2 ==
  en_m : Inport
  iread : Inport  Port=2
  iwrite : Inport  Port=3
  Compare To Constant1 : simulink/Logic and Bit Operations/Compare To Constant  relop===  const=4095  OutDataTypeStr=boolean
  RADDR_H1 : hdlsllib/HDL Operations/HDL Counter  CountType=Free running  CountInit=0  CountStep=1  CountMax=100  CountFromType=Initial value  CountFrom=0  CountResetPort=on  CountLoadPort=off  CountEnbPort=on  CountDirPort=off  CountDataType=Unsigned  CountWordLen=12  CountFracLen=0  CountSampTime=1
  Read_Write_SM1_patched_1 : State Transition Table  TreatAsAtomicUnit=on
  WADDR_H1 : hdlsllib/HDL Operations/HDL Counter  CountType=Free running  CountInit=0  CountStep=1  CountMax=100  CountFromType=Initial value  CountFrom=0  CountResetPort=on  CountLoadPort=off  CountEnbPort=on  CountDirPort=off  CountDataType=Unsigned  CountWordLen=12  CountFracLen=0  CountSampTime=1
  we : Outport
  ord_addr_H : Outport  Port=2
  owr_addr_H : Outport  Port=3
  oflag : Outport  Port=4
  wires:
  iwrite/1 -> Read_Write_SM1_patched_1/3(write)
  Read_Write_SM1_patched_1/3(enb_r) -> RADDR_H1/2
  iread/1 -> Read_Write_SM1_patched_1/2(read)
  Read_Write_SM1_patched_1/2(rst_r) -> RADDR_H1/1
  Read_Write_SM1_patched_1/5(enb_w) -> WADDR_H1/2
  en_m/1 -> Read_Write_SM1_patched_1/1(en_m)
  Read_Write_SM1_patched_1/4(rst_w) -> WADDR_H1/1
  Compare To Constant1/1 -> oflag/1
  WADDR_H1/1 -> owr_addr_H/1
  Read_Write_SM1_patched_1/1(we) -> we/1
  RADDR_H1/1 -> Compare To Constant1/1, ord_addr_H/1

== system MOSSE_HDL_final/HDL_CODER_Subsystem/SM_memory/SM_temp_G_F ==
  en_m : Inport
  iread : Inport  Port=2
  iwrite : Inport  Port=3
  RDADDR_H_n : hdlsllib/HDL Operations/HDL Counter  CountType=Free running  CountInit=0  CountStep=1  CountMax=100  CountFromType=Initial value  CountFrom=0  CountResetPort=on  CountLoadPort=off  CountEnbPort=on  CountDirPort=off  CountDataType=Unsigned  CountWordLen=12  CountFracLen=0  CountSampTime=1
  Read_Write_SM1_patched_2 : State Transition Table  TreatAsAtomicUnit=on
  WRADDR_H_n : hdlsllib/HDL Operations/HDL Counter  CountType=Free running  CountInit=0  CountStep=1  CountMax=100  CountFromType=Initial value  CountFrom=0  CountResetPort=on  CountLoadPort=off  CountEnbPort=on  CountDirPort=off  CountDataType=Unsigned  CountWordLen=12  CountFracLen=0  CountSampTime=1
  owr_addr : Outport
  we : Outport  Port=2
  ord_addr : Outport  Port=3
  wires:
  WRADDR_H_n/1 -> owr_addr/1
  iread/1 -> Read_Write_SM1_patched_2/2(read)
  Read_Write_SM1_patched_2/1(we) -> we/1
  iwrite/1 -> Read_Write_SM1_patched_2/3(write)
  en_m/1 -> Read_Write_SM1_patched_2/1(en_m)
  RDADDR_H_n/1 -> ord_addr/1
  Read_Write_SM1_patched_2/2(rst_r) -> RDADDR_H_n/1
  Read_Write_SM1_patched_2/3(enb_r) -> RDADDR_H_n/2
  Read_Write_SM1_patched_2/4(rst_w) -> WRADDR_H_n/1
  Read_Write_SM1_patched_2/5(enb_w) -> WRADDR_H_n/2

== system MOSSE_HDL_final/HDL_CODER_Subsystem/SM_memory/im_RAM_STM ==
  en_m : Inport
  read_m : Inport  Port=2
  write_m : Inport  Port=3
  ADDR_iPix1 : hdlsllib/HDL Operations/HDL Counter  CountType=Free running  CountInit=0  CountStep=1  CountMax=100  CountFromType=Initial value  CountFrom=0  CountResetPort=on  CountLoadPort=off  CountEnbPort=on  CountDirPort=off  CountDataType=Unsigned  CountWordLen=14  CountFracLen=0  CountSampTime=1
  Compare To Constant : simulink/Logic and Bit Operations/Compare To Constant  relop===  const=16383  OutDataTypeStr=boolean
  Delay2 : Delay  DelayLength=1  InitialCondition=0
  Read_Write_patched_2 : State Transition Table  TreatAsAtomicUnit=on
  Terminator1 : Terminator
  Terminator2 : Terminator
  ocount : Outport
  we_m : Outport  Port=2
  oflag : Outport  Port=3
  wires:
  Compare To Constant/1 -> Delay2/1
  write_m/1 -> Read_Write_patched_2/3(write)
  Read_Write_patched_2/1(we) -> we_m/1
  read_m/1 -> Read_Write_patched_2/2(read)
  en_m/1 -> Read_Write_patched_2/1(en_m)
  ADDR_iPix1/1 -> ocount/1, Compare To Constant/1
  Read_Write_patched_2/4(rst_w) -> ADDR_iPix1/1
  Read_Write_patched_2/5(enb_w) -> ADDR_iPix1/2
  Read_Write_patched_2/2(rst_r) -> Terminator1/1
  Read_Write_patched_2/3(enb_r) -> Terminator2/1
  Delay2/1 -> oflag/1

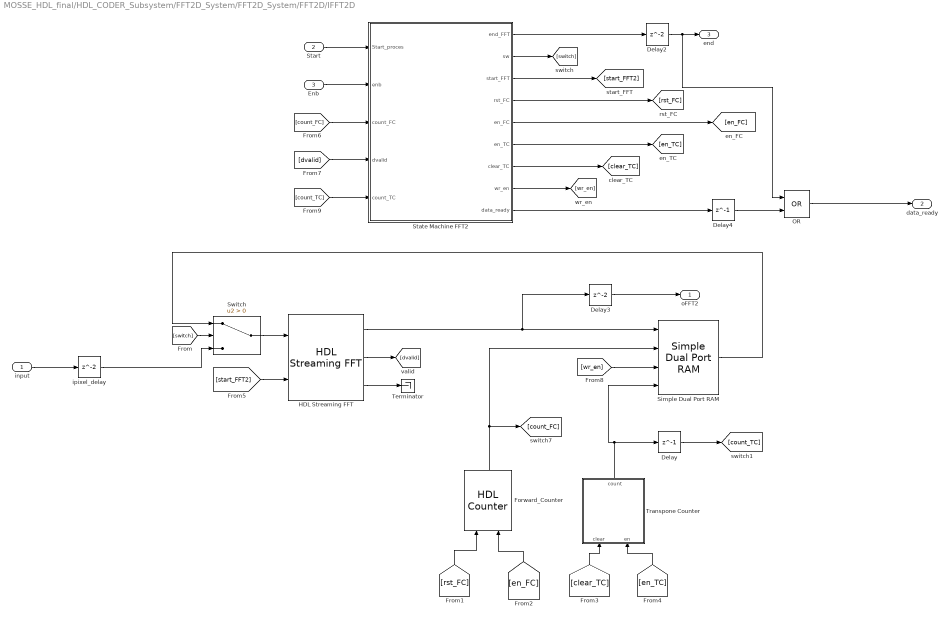
== system MOSSE_HDL_final/HDL_CODER_Subsystem/FFT2D_System/FFT2D_System/FFT2D/IFFT2D ==
  input : Inport
  Start : Inport  Port=2
  Enb : Inport  Port=3
  Delay : Delay  DelayLength=1  InitialCondition=0
  Delay2 : Delay  InitialCondition=0
  Delay3 : Delay  InitialCondition=0
  Delay4 : Delay  DelayLength=1  InitialCondition=0
  Forward_Counter : hdlsllib/HDL Operations/HDL Counter  CountType=Free running  CountInit=0  CountStep=1  CountMax=4095  CountFromType=Initial value  CountFrom=0  CountResetPort=on  CountLoadPort=off  CountEnbPort=on  CountDirPort=off  CountDataType=Unsigned  CountWordLen=12  CountFracLen=0  CountSampTime=1
  HDL Streaming FFT : hdldemolib/HDL Streaming FFT  N=64  rnd=Floor  sat=Wrap  sinemode=Same word length as input  sineWL=16  prodmode=Same as input  prodWL=32  prodFL=23  accumode=Same as input  accuWL=32  accuFL=0  outputmode=Same as input  outputWL=16  outputFL=8  isBitReversed=off  dispDelay=on
  OR : Logic  Operator=OR  IconShape=distinctive  AllPortsSameDT=off  OutDataTypeStr=boolean
  Simple Dual Port RAM : hdlsllib/HDL Operations/Simple Dual Port RAM  ram_size=12
  State Machine FFT2 : State Transition Table  TreatAsAtomicUnit=on
      settings: RTWSystemCode=Inline
  Switch : Switch  Criteria=u2 > Threshold  SampleTime=1
  Terminator : Terminator
  Transpone Counter : MATLAB Function
  ipixel_delay : Delay  InitialCondition=0  SampleTime=1
  oFFT2 : Outport
  data_ready : Outport  Port=2  OutDataTypeStr=boolean
  end : Outport  Port=3  OutDataTypeStr=boolean
  wires:
  HDL Streaming FFT/3 -> Terminator/1
  ipixel_delay/1 -> Switch/3
  HDL Streaming FFT/1 -> Delay3/1, Simple Dual Port RAM/1
  Switch/1 -> HDL Streaming FFT/1
  input/1 -> ipixel_delay/1
  State Machine FFT2/1(end_FFT) -> Delay2/1
  [switch] -> Switch/2
  State Machine FFT2/2(sw) -> [switch]
  State Machine FFT2/3(start_FFT) -> [start_FFT2]
  State Machine FFT2/4(rst_FC) -> [rst_FC]
  State Machine FFT2/5(en_FC) -> [en_FC]
  State Machine FFT2/6(en_TC) -> [en_TC]
  State Machine FFT2/7(clear_TC) -> [clear_TC]
  State Machine FFT2/8(wr_en) -> [wr_en]
  Start/1 -> State Machine FFT2/1(Start_proces)
  Enb/1 -> State Machine FFT2/2(enb)
  [clear_TC] -> Transpone Counter/1(clear)
  [en_TC] -> Transpone Counter/2(en)
  [start_FFT2] -> HDL Streaming FFT/2
  HDL Streaming FFT/2 -> [dvalid]
  [count_FC] -> State Machine FFT2/3(count_FC)
  [dvalid] -> State Machine FFT2/4(dvalid)
  [wr_en] -> Simple Dual Port RAM/3
  Forward_Counter/1 -> [count_FC], Simple Dual Port RAM/2
  [en_FC] -> Forward_Counter/2
  [rst_FC] -> Forward_Counter/1
  Simple Dual Port RAM/1 -> Switch/1
  [count_TC] -> State Machine FFT2/5(count_TC)
  Delay/1 -> [count_TC]
  Transpone Counter/1(count) -> Simple Dual Port RAM/4, Delay/1
  Delay2/1 -> OR/1, end/1
  Delay3/1 -> oFFT2/1
  Delay4/1 -> OR/2
  State Machine FFT2/9(data_ready) -> Delay4/1
  OR/1 -> data_ready/1

== matlab function HDL_CODER_Subsystem/psr_code_subsys/Compute_PSR_code ==
  data: counter output double; enb input double; rst input double; max_index output double; max_value output double; mean_value output double; std_value output double; mean_finish output double; psr_finish output double; idata input double; count_std_enb input double
function [counter, max_index, max_value, mean_value, std_value, mean_finish, psr_finish]  = psr(enb, rst, idata, count_std_enb)

numtype_idata = numerictype(1,16,0);
numtype_ind = numerictype(0,13,0);
numtype_temp = numerictype(1,44,0);
numtype_bool = numerictype(0,1,0);

numtype_fm = fimath('OverflowMode', 'saturate', 'RoundMode', 'zero');
persistent max_val max_ind temp mean_val std_val count max_mean_flag std_flag psr_flag mean_end psr_end

if isempty(max_val)
    max_val = fi(0, numtype_idata, numtype_fm);
end

if isempty(max_ind)
    max_ind = fi(0, numtype_ind, numtype_fm);
end

if isempty(count)
    count = fi(0, numtype_ind, numtype_fm);
end

if isempty(count_std_enb)
    count_std_enb = fi(0, numtype_bool, numtype_fm);
end

if isempty(temp)
    temp = fi(0, numtype_temp, numtype_fm);
end

if isempty(mean_val)
    mean_val = fi(0, numtype_idata, numtype_fm);
end

if isempty(std_val)
    std_val = fi(0, numtype_temp, numtype_fm);
end

if isempty(max_mean_flag)
    max_mean_flag = fi(0, numtype_bool, numtype_fm);
end

if isempty(std_flag)
    std_flag = fi(0, numtype_bool, numtype_fm);
end

if isempty(psr_flag)
    psr_flag = fi(0, numtype_bool, numtype_fm);
end

if isempty(mean_end)
    mean_end = fi(0, numtype_bool, numtype_fm);
end

if isempty(psr_end)
    psr_end = fi(0, numtype_bool, numtype_fm);
end

if rst
    max_val = fi(0, numtype_idata, numtype_fm);
    max_ind = fi(0, numtype_ind, numtype_fm);
    count = fi(0, numtype_ind, numtype_fm);
    temp = fi(0, numtype_temp, numtype_fm);
    mean_val = fi(0, numtype_idata, numtype_fm);
    std_val = fi(0, numtype_temp, numtype_fm);
    max_mean_flag = fi(1, numtype_bool, numtype_fm);
    std_flag = fi(0, numtype_bool, numtype_fm);
    psr_flag = fi(0, numtype_bool, numtype_fm);
    mean_end = fi(0, numtype_bool, numtype_fm);
    psr_end = fi(0, numtype_bool, numtype_fm);
    
elseif enb
    if max_mean_flag
        if idata > max_val
            max_val = fi(idata, numtype_idata, numtype_fm);
            max_ind = fi(count, numtype_ind, numtype_fm);
        end
        temp = fi(temp + idata, numtype_temp, numtype_fm);
        count = fi(count + 1, numtype_ind, numtype_fm);
        if count > 4096
            mean_val = fi(bitshift(temp, -12), numtype_idata, numtype_fm);
            temp = fi(0, numtype_temp, numtype_fm);
            count = fi(0, numtype_ind, numtype_fm);
            max_mean_flag = fi(0, numtype_bool, numtype_fm);
            std_flag = fi(1, numtype_bool, numtype_fm);
            mean_end = fi(1, numtype_bool, numtype_fm);
        end
    elseif count_std_enb
        if std_flag
            temp = fi((temp + (idata - mean_val)*(idata - mean_val)), numtype_temp, numtype_fm);
            count = fi(count + 1, numtype_ind, numtype_fm);
            if count > 4096        
                std_val = fi(bitshift(temp, -12), numtype_temp, numtype_fm);
                count = fi(0, numtype_ind, numtype_fm);
                std_flag = fi(0, numtype_bool, numtype_fm);
                psr_flag = fi(1, numtype_bool, numtype_fm);
            end
        elseif psr_flag
            count = fi(count + 1, numtype_ind, numtype_fm);
            if count > 6
                count = fi(0, numtype_ind, numtype_fm);
                psr_end = fi(1, numtype_bool, numtype_fm);
                psr_flag = fi(0, numtype_bool, numtype_fm);
            end
        end
    end       
end

counter = count;
max_index = max_ind;
max_value = max_val;
mean_value = mean_val;
std_value = std_val;
mean_finish = mean_end;
psr_finish = psr_end;

end

== matlab function HDL_CODER_Subsystem/FFT2D_System/FFT2D_System/FFT2D//IFFT2D/Transpone Counter ==
  data: count output fixdt(0,12,0); clear input double; en input double
function count  = count(clear, en)


result_nt = numerictype(0,12,0);
count_nt = numerictype(0,6,0);

result_fm = fimath('OverflowMode', 'saturate', 'RoundMode', 'floor');
n = fi(64, 0,7,0, result_fm);
persistent count_reg column row

if isempty(count_reg)
    count_reg = fi(0, result_nt, result_fm);
end

if isempty(column)
    column = fi(0, count_nt, result_fm);
end

if isempty(row)
    row = fi(0, count_nt, result_fm);
end


if clear
    row = fi(0, count_nt, result_fm);
    column = fi(0, count_nt, result_fm);
    count_reg = fi(0, result_nt, result_fm);
elseif en
     
     if (column == (n-1))
         if(row ~= (n-1))
             inc_r = row + fi(1, count_nt, result_fm);
             row = fi(inc_r, count_nt, result_fm);
         else row = fi(0, count_nt, result_fm);
             
         end
         column = fi(0, count_nt, result_fm);
     else
         inc_c = column + fi(1, count_nt, result_fm);
         column = fi(inc_c, count_nt, result_fm);
     end
     count_reg = fi(column*n + row, result_nt, result_fm);
end

count = count_reg;

end

== stateflow chart HDL_CODER_Subsystem/SM_memory/SM_H_RAM/Read_Write_SM1_patched_2 ==
  settings: executeAtInitialization=1
  state state2
    entry:
    we = false;
    rst_r = false;
    rst_w = false;
    enb_w = false;
    enb_r = false;
  state state1
    entry:
    we = false;
    rst_r = true;
    enb_r = false;
    rst_w = true;
  state state3
    entry:
    we = false;
    rst_r = false;
    enb_r = true;
    rst_w = false;
    enb_w = false;
  state state4
    entry:
    we = true;
    rst_w = false;
    enb_w = true;
    rst_r = false;
    enb_r = false;
  state1 -> (junction 65) [order 2]
  (junction 65) -> state1
  (default) -> state1
  (junction 66) -> state1
  (junction 71) -> (junction 66)
  state1 -> state2 [order 1] : [en_m == true]
  state2 -> state1 [order 4] : [en_m == false]
  state2 -> (junction 67) [order 3] : [read == false && write == false && en_m == true]
  (junction 67) -> state2
  state2 -> state3 [order 1] : [read == true && write == false && en_m == true]
  (junction 68) -> state2
  (junction 73) -> (junction 68)
  state2 -> (junction 69) [order 2] : [read == false && write == true && en_m == true]
  (junction 69) -> (junction 74)
  state3 -> state2 [order 3] : [read == false && write == false && en_m == true]
  state3 -> (junction 70) [order 1] : [read == true && en_m == true]
  (junction 70) -> state3
  state3 -> state4 [order 2] : [read == false && write == true && en_m == true]
  state3 -> (junction 71) [order 4] : [en_m == false]
  (junction 75) -> (junction 71)
  state4 -> state3 [order 2] : [read == true && write == false && en_m == true]
  state4 -> (junction 72) [order 1] : [write == true && en_m == true]
  (junction 72) -> state4
  state4 -> (junction 73) [order 3] : [read == false && write == false && en_m == true]
  (junction 74) -> state4
  state4 -> (junction 75) [order 4] : [en_m == false]
  data: en_m input boolean; we output boolean; rst_r output boolean; enb_r output boolean; read input boolean; write input boolean; rst_w output boolean; enb_w output boolean

== stateflow chart HDL_CODER_Subsystem/FFT2D_System/FFT2D_System/FFT2D//IFFT2D/State Machine FFT2 ==
  settings: executeAtInitialization=1
  state state1
    entry:
    en_FC = false;
    clear_TC = true;
    en_TC = false;
    start_FFT = false;
    wr_en = false;
  state Wait_start
    entry: rst_FC = true;
    en_FC = false;
    clear_TC = true;
    en_TC = false;
    start_FFT = false;
    wr_en = false;
    sw = false;
    end_FFT = false;
    data_ready = false;
  state state2
    entry: start_FFT = true;
    rst_FC = false;
  state state3
    entry: wr_en = true;
    en_FC = true;
    start_FFT = false;
  state state4
    entry: wr_en = true;
    en_FC = true;
    start_FFT = true;
  state state5
    entry: rst_FC = false;
    en_FC = false;
    wr_en = true;
    start_FFT = false
  state state6
    entry: rst_FC = true;
    en_FC = false;
    wr_en = false;
    start_FFT = true;
    sw = true;
  state state7
    entry: en_TC = true;
    clear_TC = false;
  state state8
    entry: rst_FC = false;
    en_FC = true;
    data_ready = true;
  state state10
    entry: end_FFT = true;
    data_ready = false;
  state state9
    entry: start_FFT = false;
    en_TC = false;
    clear_TC = true;
  Wait_start -> (junction 190) [order 2]
  (junction 190) -> Wait_start
  (default) -> Wait_start
  (junction 191) -> Wait_start
  (junction 210) -> (junction 191)
  Wait_start -> state1 [order 1] : [Start_proces == true && enb == true]
  state1 -> (junction 192) [order 1] : [enb == false && dvalid == false]
  (junction 192) -> state1
  (junction 193) -> state1
  (junction 205) -> (junction 193)
  state1 -> (junction 194) [order 3] : [enb == false && dvalid == true]
  (junction 194) -> (junction 200)
  state1 -> state2 [order 2] : [enb == true && dvalid == false]
  state1 -> (junction 195) [order 4] : [enb == true && dvalid == true]
  (junction 197) -> (junction 195)
  (junction 195) -> (junction 203)
  state2 -> state1 [order 1] : [enb == false && dvalid == false]
  state2 -> (junction 196) [order 2] : [enb == true && dvalid == false]
  (junction 196) -> state2
  state2 -> (junction 197) [order 4] : [enb == true && dvalid == true]
  state2 -> state3 [order 3] : [enb == false && dvalid == true]
  (junction 198) -> state2
  (junction 204) -> (junction 198)
  state3 -> state2 [order 2] : [enb == true && dvalid == false]
  state3 -> (junction 199) [order 3]
  (junction 199) -> state3
  state3 -> state4 [order 4] : [enb == true && dvalid == true]
  state4 -> state3 [order 3] : [enb == false && dvalid == true]
  (junction 200) -> state3
  state3 -> (junction 201) [order 1] : [count_FC == 4095]
  (junction 201) -> (junction 206)
  state4 -> (junction 202) [order 4] : [enb == true && dvalid == true]
  (junction 202) -> state4
  (junction 203) -> state4
  state4 -> (junction 204) [order 2] : [enb == true && dvalid == false]
  state4 -> (junction 205) [order 1] : [enb == false && dvalid == false]
  state5 -> state6
  (junction 206) -> state5
  state6 -> state7
  state7 -> (junction 207) [order 2]
  (junction 207) -> state7
  state7 -> state8 [order 1] : [dvalid == true]
  state8 -> (junction 208) [order 2]
  (junction 208) -> state8
  state8 -> state9 [order 1] : [count_TC == 4095]
  state9 -> (junction 209) [order 2]
  (junction 209) -> state9
  state9 -> state10 [order 1] : [count_FC == 4095]
  state10 -> (junction 210)
  data: end_FFT output boolean; sw output boolean; start_FFT output boolean; rst_FC output boolean; en_FC output boolean; en_TC output boolean; clear_TC output boolean; wr_en output boolean; Start_proces input boolean; enb input boolean; count_FC input fixdt(0,12,0); dvalid input boolean; data_ready output boolean; count_TC input fixdt(0,12,0)
